simulink model "UNO_Blink_task"  (Simulink 3.00)
settings: Solver=ode45  SolverMode=SingleTasking  StartTime=0.0  StopTime=10.0  RelTol=1e-3
libraries: genlib x4, REXduino_library x1
settings Model: Creator=Jarda  LastModifiedBy=XPMUser

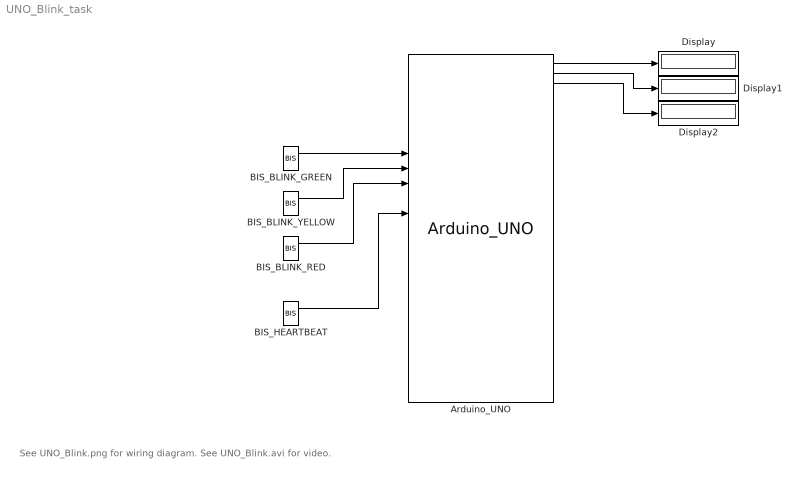
== system UNO_Blink_task ==
  note: See UNO_Blink.png for wiring diagram.
      |
      | See UNO_Blink.avi for video.
  Arduino_UNO : REXduino_library/Arduino_UNO  comPort=/dev/ttyACM0  pinmode2=1: Not connected  pinmode3=1: Not connected  pinmode4=1: Not connected  pinmode5=1: Not connected  pinmode6=1: Not connected  pinmode9=2: Digital output  pinmode10=2: Digital output  pinmode11=2: Digital output  pinmodeA0=1: Not connected  pinmodeA1=1: Not connected  pinmodeA2=1: Not connected  pinmodeA3=1: Not connected  pinmodeA4=1: Not connected  pinmodeA5=1: Not connected  usercmd=1: No data
  BIS_BLINK_GREEN : genlib/BIS  Y0=off  t1=0.5  t2=1  t3=0  t4=4  t5=5  t6=6  t7=7  t8=8  RPT=on  bEdit=off
  BIS_BLINK_RED : genlib/BIS  Y0=off  t1=2  t2=4  t3=0  t4=4  t5=5  t6=6  t7=7  t8=8  RPT=on  bEdit=off
  BIS_BLINK_YELLOW : genlib/BIS  Y0=off  t1=1  t2=2  t3=0  t4=4  t5=5  t6=6  t7=7  t8=8  RPT=on  bEdit=off
  BIS_HEARTBEAT : genlib/BIS  Y0=off  t1=0.7  t2=0.8  t3=0.9  t4=1.0  t5=0  t6=6  t7=7  t8=8  RPT=on  bEdit=off
  Display : Display
      settings: Format=Best fit
  Display1 : Display
      settings: Format=Best fit
  Display2 : Display
      settings: Format=Best fit
  wires:
  Arduino_UNO/1 -> Display/1
  Arduino_UNO/2 -> Display1/1
  Arduino_UNO/3 -> Display2/1
  BIS_BLINK_GREEN/1 -> Arduino_UNO/6
  BIS_BLINK_RED/1 -> Arduino_UNO/8
  BIS_BLINK_YELLOW/1 -> Arduino_UNO/7
  BIS_HEARTBEAT/1 -> Arduino_UNO/10
